simulink model "TORA_Non_Linear"  (R2019b)
settings: Solver=VariableStepAuto  StartTime=0.0  StopTime=10.0  RelTol=1e-3
values from neighbouring files (symbols this model uses):
  A = double(subs(JacobianA, vars, x_bar))    [TORA_math2.m]
  B = double(subs(jacobianB, vars, x_bar))    [TORA_math2.m]
  C = [1 0 0 0 ... (first row only)    [TORA_math2.m]
  J = 0.0002175    [TORA_math2.m]    (also in TORA_math3.m; main.m)
  k = 186.3    [TORA_math2.m]    (also in TORA_math3.m; main.m)
  L = 1    [TORA_math3.m]    (also in main.m)
  M = 1.3608    [TORA_math2.m]    (also in TORA_math3.m; main.m)
  m = 0.096    [TORA_math2.m]    (also in TORA_math3.m; main.m)
  x0 = [0 0 0.01 0.01]'    [TORA_math2.m]
  x_bar = [0 0 0 0]    [TORA_math2.m]
undefined symbols (not defined in the file or in its folder): Boolean_Controller, G, L_new, stateEstimates
settings Model: Creator=don  LastModifiedBy=don

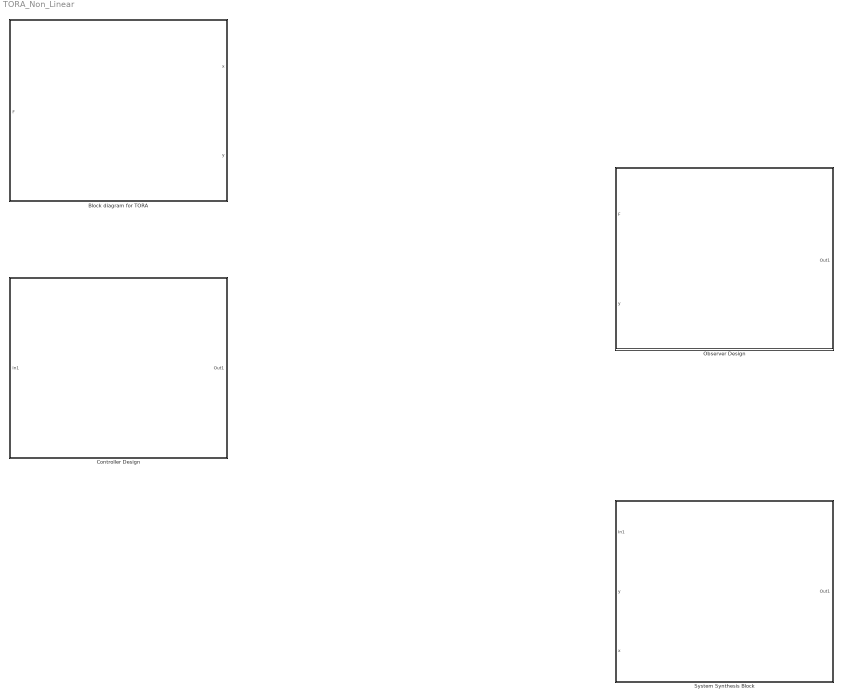
== system TORA_Non_Linear ==
  Block diagram for TORA : Subsystem
  "Controller Design " : Subsystem
  Observer Design : Subsystem
  System Synthesis Block : Subsystem

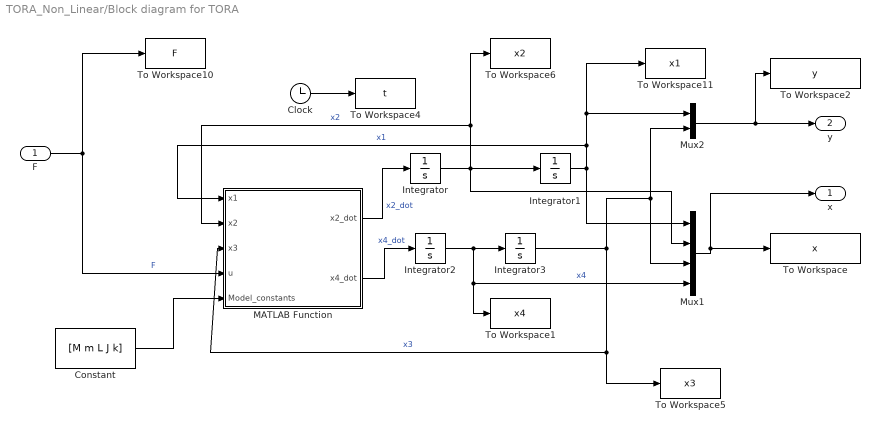
== system TORA_Non_Linear/Block diagram for TORA ==
  F : Inport
  Clock : Clock
  Constant : Constant  Value=[M m L J k]
  Integrator : Integrator  InitialCondition=x0(2)
  Integrator1 : Integrator  InitialCondition=x0(1)
  Integrator2 : Integrator  InitialCondition=x0(4)
  Integrator3 : Integrator  InitialCondition=x0(3)
  MATLAB Function : MATLAB Function  TreatAsAtomicUnit=on
  Mux1 : Mux
  Mux2 : Mux  Inputs=2
  To Workspace : ToWorkspace  VariableName=x  SampleTime=-1
  To Workspace1 : ToWorkspace  VariableName=x4  SampleTime=-1
  To Workspace10 : ToWorkspace  VariableName=F  SampleTime=-1
  To Workspace11 : ToWorkspace  VariableName=x1  SampleTime=-1
  To Workspace2 : ToWorkspace  VariableName=y  SampleTime=-1
  To Workspace4 : ToWorkspace  VariableName=t  SampleTime=-1
  To Workspace5 : ToWorkspace  VariableName=x3  SampleTime=-1
  To Workspace6 : ToWorkspace  VariableName=x2  SampleTime=-1
  x : Outport  VectorParamsAs1DForOutWhenUnconnected=off
  y : Outport  Port=2  VectorParamsAs1DForOutWhenUnconnected=off
  wires:
  F/1 -> MATLAB Function/4(u), To Workspace10/1  "F"
  Integrator1/1 -> To Workspace11/1, Mux2/1, MATLAB Function/1(x1), Mux1/1  "x1"
  Mux1/1 -> x/1, To Workspace/1
  Clock/1 -> To Workspace4/1
  Mux2/1 -> y/1, To Workspace2/1
  Integrator/1 -> Mux1/2, To Workspace6/1, MATLAB Function/2(x2), Integrator1/1  "x2"
  Constant/1 -> MATLAB Function/5(Model_constants)
  MATLAB Function/1(x2_dot) -> Integrator/1  "x2_dot"
  Integrator2/1 -> To Workspace1/1, Mux1/4, Integrator3/1  "x4"
  MATLAB Function/2(x4_dot) -> Integrator2/1  "x4_dot"
  Integrator3/1 -> To Workspace5/1, MATLAB Function/3(x3), Mux2/2, Mux1/3  "x3"

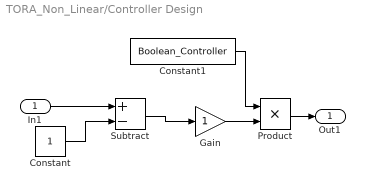
== system TORA_Non_Linear/Controller Design  ==
  In1 : Inport
  Constant : Constant
  Constant1 : Constant  Value=Boolean_Controller
  Gain : Gain
  Product : Product
  Subtract : Sum  Inputs=+-
  Out1 : Outport
  wires:
  Subtract/1 -> Gain/1
  Gain/1 -> Product/2
  Product/1 -> Out1/1
  Constant/1 -> Subtract/2
  In1/1 -> Subtract/1
  Constant1/1 -> Product/1

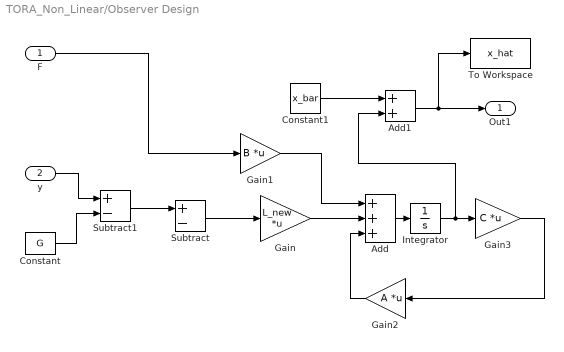
== system TORA_Non_Linear/Observer Design ==
  F : Inport
  y : Inport  Port=2
  Add : Sum  Inputs=+++
  Add1 : Sum
  Constant : Constant  Value=G
  Constant1 : Constant  Value=x_bar
  Gain : Gain  Gain=L_new  Multiplication=Matrix(K*u)
  Gain1 : Gain  Gain=B  Multiplication=Matrix(K*u)
  Gain2 : Gain  Gain=A  Multiplication=Matrix(K*u)
  Gain3 : Gain  Gain=C  Multiplication=Matrix(K*u)
  Integrator : Integrator
  Subtract : Sum  Inputs=+-
  Subtract1 : Sum  Inputs=+-
  To Workspace : ToWorkspace  VariableName=x_hat  SampleTime=-1
  Out1 : Outport
  wires:
  Constant/1 -> Subtract1/2
  y/1 -> Subtract1/1
  F/1 -> Gain1/1
  Subtract1/1 -> Subtract/1
  Subtract/1 -> Gain/1
  Gain/1 -> Add/2
  Gain2/1 -> Add/3
  Add/1 -> Integrator/1
  Integrator/1 -> Add1/2, Gain3/1
  Gain3/1 -> Gain2/1
  Add1/1 -> To Workspace/1, Out1/1
  Constant1/1 -> Add1/1
  Gain1/1 -> Add/1

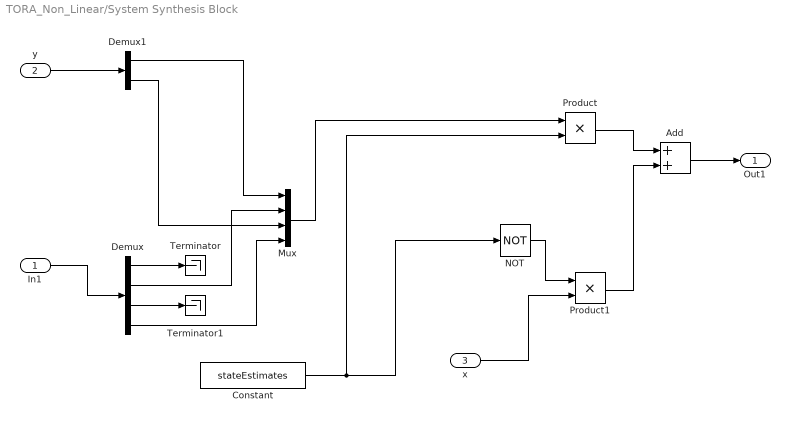
== system TORA_Non_Linear/System Synthesis Block ==
  In1 : Inport
  y : Inport  Port=2
  x : Inport  Port=3
  Add : Sum
  Constant : Constant  Value=stateEstimates
  Demux : Demux
  Demux1 : Demux  Outputs=2
  Mux : Mux
  NOT : Logic  Operator=NOT  IconShape=distinctive  AllPortsSameDT=off  OutDataTypeStr=boolean
  Product : Product
  Product1 : Product
  Terminator : Terminator
  Terminator1 : Terminator
  Out1 : Outport
  wires:
  Add/1 -> Out1/1
  y/1 -> Demux1/1
  In1/1 -> Demux/1
  Demux/1 -> Terminator/1
  Product1/1 -> Add/2
  Product/1 -> Add/1
  Demux1/1 -> Mux/1
  NOT/1 -> Product1/1
  x/1 -> Product1/2
  Demux1/2 -> Mux/3
  Demux/2 -> Mux/2
  Demux/4 -> Mux/4
  Demux/3 -> Terminator1/1
  Constant/1 -> NOT/1, Product/2
  Mux/1 -> Product/1

== matlab function TORA_Non_Linear/Block diagram for TORA/MATLAB Function ==
  data: x1 input; x2_dot output; x2 input; x3 input; u input; x4_dot output; Model_constants input
 function [x2_dot,x4_dot] = NonLinearEquations(x1,x2,x3,u,Model_constants)

%Get Model Constants:
M = Model_constants(1);
m = Model_constants(2);
J = Model_constants(3);
k = Model_constants(4);
L = Model_constants(5);

%x2_dot equation
x2_dot = (((m+M)*u)-(m*L*cos(x1)*(m*L*(x2^2)*sin(x1)-(k*(x3)))))/((J+(m*(L^2))*(m+M))-((m^2)*(L^2)*cos(x1)^2));

%x4_dot equation
x4_dot = ((-m*L*u*cos(x1))+(J+(m*(L^2)))*(m*L*(x2^2)*sin(x1)-k*(x3)))/((J+(m*(L^2))*(m+M))-((m^2)*L^2*cos(x1)^2));

end
